simulink model "simulink_act1_ses1_grupo1_exp1_act3"  (R2021b)
settings: Solver=ode2  StartTime=0.0  StopTime=10.0  FixedStep=0.01  RelTol=1e-3
model workspace (MAT data in the model file):
  y = 0
  y_0 = 0
settings Model: Creator=LABCONTROL1  LastModifiedBy=LABCONTROL1
settings DataIOCC: ReturnWorkspaceOutputs=off

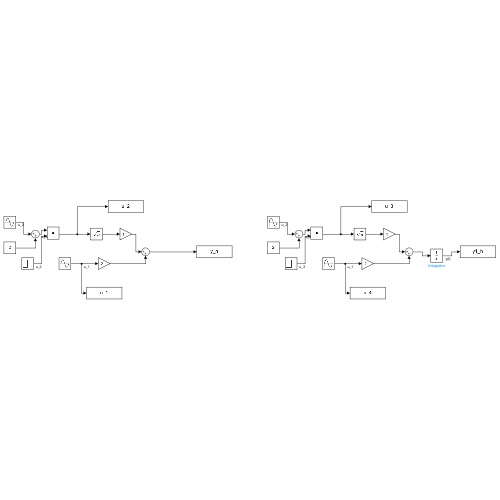
[thumbnail: Simulink's stored preview of the top-level diagram]
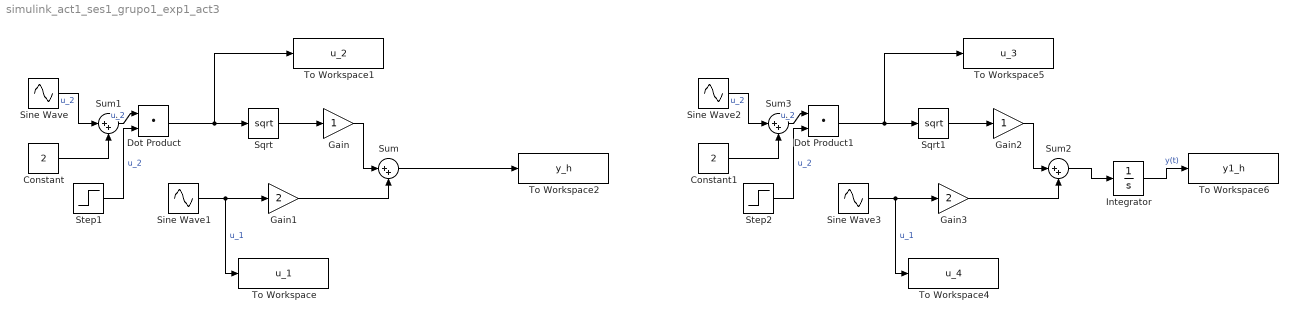
== system simulink_act1_ses1_grupo1_exp1_act3 ==
  Constant : Constant  Value=2
  Constant1 : Constant  Value=2
  Dot Product : DotProduct  InputSameDT=on  OutDataTypeStr=Inherit: Inherit via internal rule
  Dot Product1 : DotProduct  InputSameDT=on  OutDataTypeStr=Inherit: Inherit via internal rule
  Gain : Gain
  Gain1 : Gain  Gain=2
  Gain2 : Gain
  Gain3 : Gain  Gain=2
  Integrator : Integrator
  Sine Wave : Sin  Amplitude=1.5  Frequency=10  SampleTime=0
  Sine Wave1 : Sin  Frequency=100  SampleTime=0
  Sine Wave2 : Sin  Amplitude=1.5  Frequency=10  SampleTime=0
  Sine Wave3 : Sin  Frequency=100  SampleTime=0
  Sqrt : Sqrt  SaturateOnIntegerOverflow=on
  Sqrt1 : Sqrt  SaturateOnIntegerOverflow=on
  Step1 : Step  SampleTime=0
  Step2 : Step  SampleTime=0
  Sum{,1..3} (4 alike) : Sum  Inputs=|++
  To Workspace : ToWorkspace  VariableName=u_1  SampleTime=0.5
      settings: Save2DSignal=2-D array (concatenate along first dimension)
  To Workspace1 : ToWorkspace  VariableName=u_2  SampleTime=0.5
      settings: Save2DSignal=2-D array (concatenate along first dimension)
  To Workspace2 : ToWorkspace  VariableName=y_h  SampleTime=0.5
      settings: Save2DSignal=2-D array (concatenate along first dimension)
  To Workspace4 : ToWorkspace  VariableName=u_4  SampleTime=0.5
      settings: Save2DSignal=2-D array (concatenate along first dimension)
  To Workspace5 : ToWorkspace  VariableName=u_3  SampleTime=0.5
      settings: Save2DSignal=2-D array (concatenate along first dimension)
  To Workspace6 : ToWorkspace  VariableName=y1_h  SampleTime=0.5
      settings: Save2DSignal=2-D array (concatenate along first dimension)
  wires:
  Gain1/1 -> Sum/2
  Sine Wave1/1 -> To Workspace/1, Gain1/1  "u_1"
  Sum/1 -> To Workspace2/1
  Step1/1 -> Dot Product/2  "u_2"
  Sqrt/1 -> Gain/1
  Gain/1 -> Sum/1
  Sine Wave/1 -> Sum1/1  "u_2"
  Constant/1 -> Sum1/2
  Sum1/1 -> Dot Product/1  "u_2"
  Dot Product/1 -> To Workspace1/1, Sqrt/1
  Sine Wave2/1 -> Sum3/1  "u_2"
  Sum3/1 -> Dot Product1/1  "u_2"
  Constant1/1 -> Sum3/2
  Gain2/1 -> Sum2/1
  Step2/1 -> Dot Product1/2  "u_2"
  Gain3/1 -> Sum2/2
  Dot Product1/1 -> To Workspace5/1, Sqrt1/1
  Sine Wave3/1 -> To Workspace4/1, Gain3/1  "u_1"
  Integrator/1 -> To Workspace6/1  "y(t)"
  Sqrt1/1 -> Gain2/1
  Sum2/1 -> Integrator/1
